simulink model "LAB_ROTORE"  (R2022b)
settings: Solver=ode4  StartTime=0.0  StopTime=100  FixedStep=0.1  RelTol=1e-3
values from neighbouring files (symbols this model uses):
  I = [Ix 0 0 ... (first row only)    [LAB_03_3_OCT_MAT_EUL_2_VERIFICATION.m]    (also in LAB_03_3_OCT_MAT_EUL_DOUBLESPIN.m = diag([Ix, Iy, Iz]); LAB_03_3_OCT_MAT_EUL_SPINAXIS.m = diag([Ix, Iy, Iz]); LAB_03_3_OCT_MAT_EUL_VECT.m; LAB_04_17_OCT_MAT_KIN.m)
  Ir = diag([0, 0, Ir_value])    [LAB_03_3_OCT_MAT_EUL_DOUBLESPIN.m]
  om_0 = [om_x0, om_y0, om_z0]    [LAB_03_3_OCT_MAT_EUL.m]    (also in LAB_03_3_OCT_MAT_EUL_2_VERIFICATION.m = [om_x0; om_y0; om_z0]; LAB_03_3_OCT_MAT_EUL_DOUBLESPIN.m = [om_x0; om_y0; om_z0]; LAB_03_3_OCT_MAT_EUL_SPINAXIS.m = [om_x0; om_y0; om_z0]; LAB_03_3_OCT_MAT_EUL_VECT.m = [om_x0; om_y0; om_z0])
  om_r0 = [0, 0, 2*pi]    [LAB_03_3_OCT_MAT_EUL_DOUBLESPIN.m]
  Tw = [0; 0; 0]    [LAB_03_3_OCT_MAT_EUL_DOUBLESPIN.m]
libraries: matrix_library x1
settings Model: Creator=maria  LastModifiedBy=maria

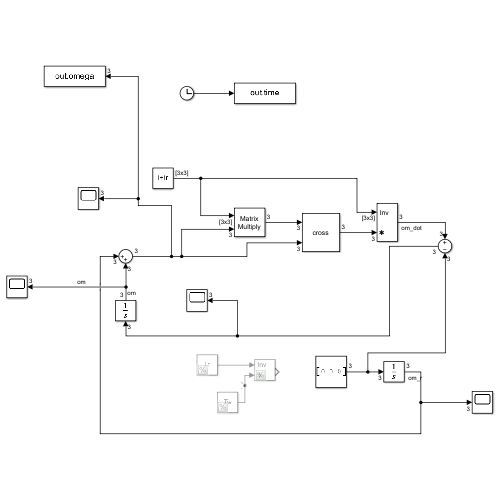
[thumbnail: Simulink's stored preview of the top-level diagram]
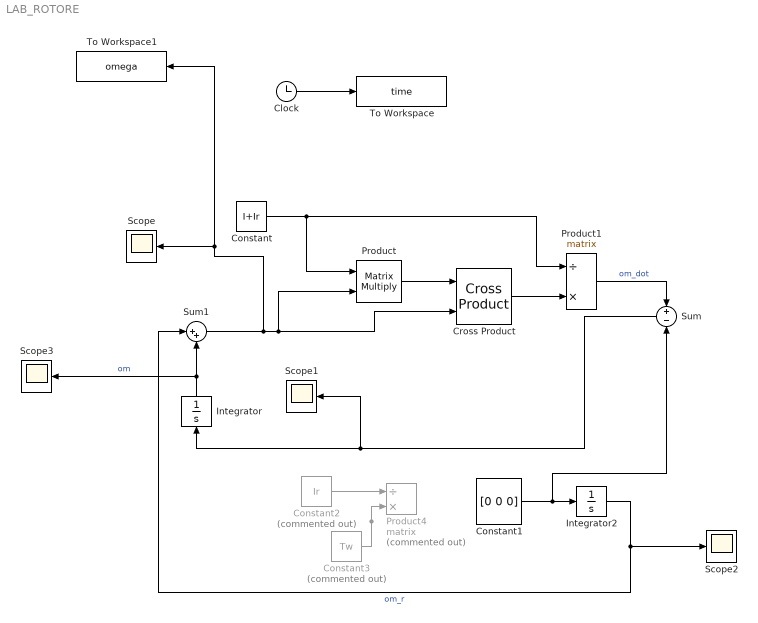
== system LAB_ROTORE ==
  Clock : Clock
  Constant : Constant  Value=I+Ir
  Constant1 : Constant  Value=[0 0 0]
  Constant2 : Constant  Commented=on  Value=Ir
  Constant3 : Constant  Commented=on  Value=Tw
  Cross Product : matrix_library/Cross Product
  Integrator : Integrator  InitialCondition=om_0
  Integrator2 : Integrator  InitialCondition=om_r0
  Product : Product  Multiplication=Matrix(*)
  Product1 : Product  Inputs=/*  Multiplication=Matrix(*)
  Product4 : Product  Commented=on  Inputs=/*  Multiplication=Matrix(*)
  Scope{,1..3} (4 alike) : Scope
  Sum : Sum  Inputs=+-
  Sum1 : Sum  Inputs=|++
  To Workspace : ToWorkspace  VariableName=time  SaveFormat=Timeseries  SampleTime=-1
  To Workspace1 : ToWorkspace  VariableName=omega  SaveFormat=Timeseries  SampleTime=-1
  wires:
  Product1/1 -> Sum/1  "om_dot"
  Sum/1 -> Scope1/1, Integrator/1
  Constant3/1 -> Product4/2
  Product/1 -> Cross Product/1
  Constant/1 -> Product/1, Product1/1
  Integrator/1 -> Scope3/1, Sum1/2  "om"
  Cross Product/1 -> Product1/2
  Clock/1 -> To Workspace/1
  Constant2/1 -> Product4/1
  Integrator2/1 -> Scope2/1, Sum1/1  "om_r"
  Sum1/1 -> To Workspace1/1, Scope/1, Product/2, Cross Product/2
  Constant1/1 -> Sum/2, Integrator2/1
